simulink model "SVPWM_Combined"  (R2018b)
settings: Solver=FixedStepAuto  StartTime=0.0  StopTime=2000e-3  FixedStep=5e-7  RelTol=1e-3
libraries: powerlib x30, powerlib_meascontrol x5
settings Model: Creator=seogan  LastModifiedBy=Lenovo

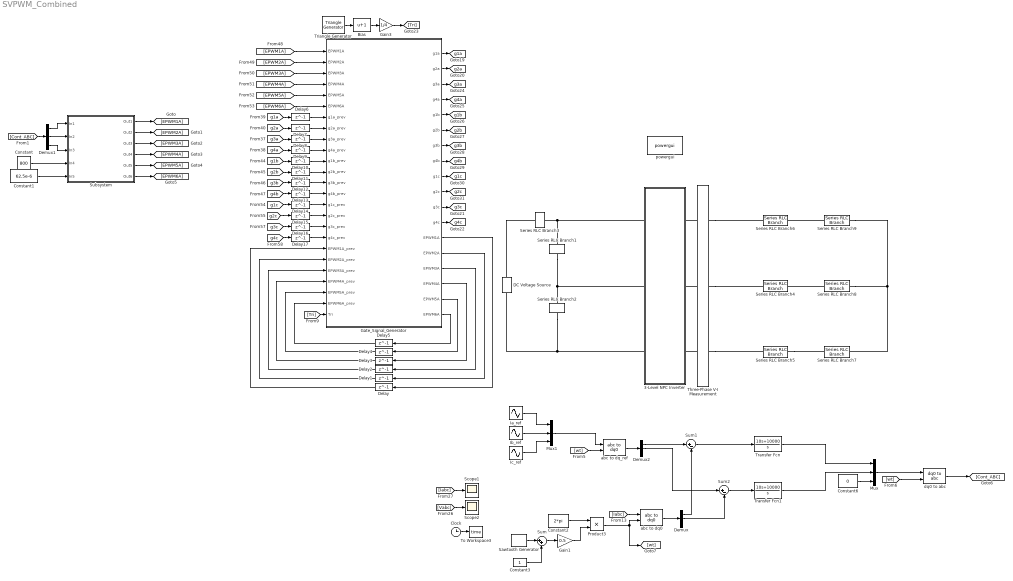
== system SVPWM_Combined ==
  3-Level NPC Inverter : Subsystem
  Bias : Bias  Bias=1
  Clock : Clock
  Constant : Constant  Value=800
  Constant1 : Constant  Value=62.5e-6
  Constant2 : Constant  Value=2*pi
  Constant3 : Constant
  Constant6 : Constant  Value=0
  DC Voltage Source : powerlib/Electrical Sources/DC Voltage Source  Amplitude=800  Measurements=None
  Delay{,1..17} (18 alike) : Delay  DelayLength=1
  Demux : Demux  Outputs=3
  Demux1 : Demux  Outputs=3
  Demux2 : Demux  Outputs=3
  Gain1 : Gain  Gain=0.5
  Gain3 : Gain  Gain=1/4
  Gate_Signal_Generator : MATLAB Function  TreatAsAtomicUnit=on
  Ia_ref : Sin  Amplitude=87.4  Frequency=50*2*pi  Phase=-62*pi/180  SampleTime=0
  Ib_ref : Sin  Amplitude=87.4  Frequency=50*2*pi  Phase=-62*pi/180-2*pi/3  SampleTime=0
  Ic_ref : Sin  Amplitude=87.4  Frequency=50*2*pi  Phase=-62*pi/180-4*pi/3  SampleTime=0
  Mux : Mux  Inputs=3
  Mux1 : Mux  Inputs=3
  Product3 : Product
  Sawtooth Generator : powerlib_meascontrol/Pulse & Signal Generators/Sawtooth Generator  Freq=50  Phase=0  Ts=5e-7
      settings: SourceProductName=Simscape Power Systems
  Scope1 : Scope
  Scope2 : Scope
  Series RLC Branch1 : powerlib/Elements/Series RLC Branch  LConnTagsString=__new0  RConnTagsString=__new0  BranchType=C  Resistance=1e-3  Inductance=1e-3  SetiL0=off  InitialCurrent=0  Capacitance=500e-6  Setx0=on  InitialVoltage=800/2  Measurements=Branch voltage
  Series RLC Branch2 : powerlib/Elements/Series RLC Branch  LConnTagsString=__new0  RConnTagsString=__new0  BranchType=C  Resistance=1e-3  Inductance=1e-3  SetiL0=off  InitialCurrent=0  Capacitance=500e-6  Setx0=on  InitialVoltage=800/2  Measurements=None
  Series RLC Branch3 : powerlib/Elements/Series RLC Branch  LConnTagsString=__new0  RConnTagsString=__new0  BranchType=R  Resistance=1e-3  Inductance=10e-3  SetiL0=on  InitialCurrent=88  Capacitance=1e-6  Setx0=off  InitialVoltage=0  Measurements=None
  Series RLC Branch4 : powerlib/Elements/Series RLC Branch  LConnTagsString=__new0  RConnTagsString=__new0  BranchType=R  Resistance=0.1  Inductance=0.6e-3  SetiL0=off  InitialCurrent=0  Capacitance=1e-6  Setx0=off  InitialVoltage=0  Measurements=None
  Series RLC Branch5 : powerlib/Elements/Series RLC Branch  LConnTagsString=__new0  RConnTagsString=__new0  BranchType=R  Resistance=0.1  Inductance=0.6e-3  SetiL0=off  InitialCurrent=0  Capacitance=1e-6  Setx0=off  InitialVoltage=0  Measurements=None
  Series RLC Branch6 : powerlib/Elements/Series RLC Branch  LConnTagsString=__new0  RConnTagsString=__new0  BranchType=R  Resistance=0.1  Inductance=0.6e-3  SetiL0=off  InitialCurrent=0  Capacitance=1e-6  Setx0=off  InitialVoltage=0  Measurements=None
  Series RLC Branch7 : powerlib/Elements/Series RLC Branch  LConnTagsString=__new0  RConnTagsString=__new0  BranchType=L  Resistance=0.1  Inductance=0.6e-3  SetiL0=off  InitialCurrent=0  Capacitance=1e-6  Setx0=off  InitialVoltage=0  Measurements=None
  Series RLC Branch8 : powerlib/Elements/Series RLC Branch  LConnTagsString=__new0  RConnTagsString=__new0  BranchType=L  Resistance=0.1  Inductance=0.6e-3  SetiL0=off  InitialCurrent=0  Capacitance=1e-6  Setx0=off  InitialVoltage=0  Measurements=None
  Series RLC Branch9 : powerlib/Elements/Series RLC Branch  LConnTagsString=__new0  RConnTagsString=__new0  BranchType=L  Resistance=0.1  Inductance=0.6e-3  SetiL0=off  InitialCurrent=0  Capacitance=1e-6  Setx0=off  InitialVoltage=0  Measurements=None
  Subsystem : Subsystem
  Sum : Sum  Inputs=|++
  Sum1 : Sum  Inputs=|+-
  Sum2 : Sum  Inputs=|+-
  Three-Phase V-I Measurement : powerlib/Measurements/Three-Phase V-I Measurement  VoltageMeasurement=phase-to-phase  SetLabelV=on  LabelV=Vabc  Vpu=off  VpuLL=off  CurrentMeasurement=yes  SetLabelI=on  LabelI=Iabc  Ipu=off  Pbase=100e6  Vbase=500e3  OutputType=Complex  PhasorSimulation=off  PSBequivalent=0
  To Workspace3 : ToWorkspace  VariableName=time  SampleTime=-1
  Transfer Fcn : TransferFcn  Numerator=[10 10000]  Denominator=[1 0]
  Transfer Fcn1 : TransferFcn  Numerator=[10 10000]  Denominator=[1 0]
  Triangle Generator : powerlib_meascontrol/Pulse & Signal Generators/Triangle Generator  Freq=16e3  Phase=0  Ts=5e-7
  abc to dq0 : powerlib_meascontrol/Transformations/abc to dq0  Alignment=90 degrees behind phase A axis
  abc to dq_ref : powerlib_meascontrol/Transformations/abc to dq0  Alignment=90 degrees behind phase A axis
  dq0 to abc : powerlib_meascontrol/Transformations/dq0 to abc  Alignment=90 degrees behind phase A axis
  powergui : powerlib/powergui  Priority=1  SimulationMode=Discrete  SampleTime=500e-9  frequency=60  Iterations=50  frequencyindice=0  Pbase=100e6  ErrMax=1e-4  UnitsV=kV  UnitsW=MW  buscounter=0  FunctionMessages=off  echomessages=off  EnableUseOfTLC=off  CurrentSourceSwitches=off  DisableSnubberDevices=off  DisableRonSwitches=off  DisableVfSwitches=off  DisplayEquations=off  SolverType=Tustin/Backward Euler (TBE)  Interpol=off  ExternalGateDelay=off  methode=off  Ts=100  x0status=blocks  SPID=off  SwTol=0  HookPort=off  RestoreLinks=warning  ResistiveCurrentMeasurement=off  Frange=[0:2:500]  Ylog=off  Xlog=on  ShowGrid=off  save=off  variable=ZData  structure=0  ZoomFFT=off  StartTime=0.0  cycles=1  DisplayStyle=1  fundamental=60  FreqAxis=off  MaxFrequency=1000  frequencyindicesteady=1  RmsSteady=1  display=off
  tag scope: g1a=global, g1b=global, g1c=global, g2a=global, g2b=global, g2c=global, g3a=global, g3b=global, g3c=global, g4a=global, g4b=global, g4c=global
  wires:
  Clock/1 -> To Workspace3/1
  Gate_Signal_Generator/8(g4b) -> [g4b]
  [EPWM3A] -> Gate_Signal_Generator/3("EPWM3A ")
  Delay2/1 -> Gate_Signal_Generator/21(EPWM3A_prev)
  Gate_Signal_Generator/5(g1b) -> [g1b]
  Gate_Signal_Generator/18(EPWM6A) -> Delay5/1
  Gain3/1 -> [Tri]
  Gate_Signal_Generator/7(g3b) -> [g3b]
  Gate_Signal_Generator/16(EPWM4A) -> Delay3/1
  Gate_Signal_Generator/15(EPWM3A) -> Delay2/1
  Gate_Signal_Generator/4(g4a) -> [g4a]
  Gate_Signal_Generator/3(g3a) -> [g3a]
  Gate_Signal_Generator/14(EPWM2A) -> Delay1/1
  [EPWM5A] -> Gate_Signal_Generator/5("EPWM5A ")
  [EPWM2A] -> Gate_Signal_Generator/2("EPWM2A ")
  [EPWM6A] -> Gate_Signal_Generator/6("EPWM6A ")
  Gate_Signal_Generator/13(EPWM1A) -> Delay/1
  [EPWM4A] -> Gate_Signal_Generator/4("EPWM4A ")
  Delay3/1 -> Gate_Signal_Generator/22(EPWM4A_prev)
  Gate_Signal_Generator/6(g2b) -> [g2b]
  [EPWM1A] -> Gate_Signal_Generator/1("EPWM1A ")
  Bias/1 -> Gain3/1
  Gate_Signal_Generator/9(g1c) -> [g1c]
  Gate_Signal_Generator/2(g2a) -> [g2a]
  Gate_Signal_Generator/11(g3c) -> [g3c]
  Delay5/1 -> Gate_Signal_Generator/24(EPWM6A_prev)
  Gate_Signal_Generator/10(g2c) -> [g2c]
  Delay4/1 -> Gate_Signal_Generator/23(EPWM5A_prev)
  Delay1/1 -> Gate_Signal_Generator/20(EPWM2A_prev)
  Gate_Signal_Generator/1(g1a) -> [g1a]
  Gate_Signal_Generator/12(g4c) -> [g4c]
  Gate_Signal_Generator/17(EPWM5A) -> Delay4/1
  Delay/1 -> Gate_Signal_Generator/19(EPWM1A_prev)
  [Tri] -> Gate_Signal_Generator/25(Tri)
  Triangle Generator/1 -> Bias/1
  Delay6/1 -> Gate_Signal_Generator/7(g1a_prev)
  [g1a] -> Delay6/1
  Delay7/1 -> Gate_Signal_Generator/8(g2a_prev)
  Delay8/1 -> Gate_Signal_Generator/9(g3a_prev)
  Delay9/1 -> Gate_Signal_Generator/10(g4a_prev)
  [g2a] -> Delay7/1
  [g3a] -> Delay8/1
  [g4a] -> Delay9/1
  Delay10/1 -> Gate_Signal_Generator/11(g1b_prev)
  Delay11/1 -> Gate_Signal_Generator/12(g2b_prev)
  Delay12/1 -> Gate_Signal_Generator/13(g3b_prev)
  Delay13/1 -> Gate_Signal_Generator/14(g4b_prev)
  [g1b] -> Delay10/1
  [g2b] -> Delay11/1
  [g3b] -> Delay12/1
  [g4b] -> Delay13/1
  Delay14/1 -> Gate_Signal_Generator/15(g1c_prev)
  Delay15/1 -> Gate_Signal_Generator/16(g2c_prev)
  Delay16/1 -> Gate_Signal_Generator/17(g3c_prev)
  Delay17/1 -> Gate_Signal_Generator/18(g4c_prev)
  [g1c] -> Delay14/1
  [g2c] -> Delay15/1
  [g3c] -> Delay16/1
  [g4c] -> Delay17/1
  [Vabc] -> Scope2/1
  [Iabc] -> Scope1/1
  Sawtooth Generator/1 -> Sum/1
  Constant3/1 -> Sum/2
  Sum/1 -> Gain1/1
  Gain1/1 -> Product3/2
  Constant2/1 -> Product3/1
  Product3/1 -> abc to dq0/2, [wt]
  Demux/1 -> Sum1/2
  Demux/2 -> Sum2/2
  Mux/1 -> dq0 to abc/1
  Constant6/1 -> Mux/3
  dq0 to abc/1 -> [Cont_ABC]
  [wt] -> abc to dq_ref/2
  Mux1/1 -> abc to dq_ref/1
  Ib_ref/1 -> Mux1/2
  Ia_ref/1 -> Mux1/1
  Ic_ref/1 -> Mux1/3
  abc to dq_ref/1 -> Demux2/1
  [wt] -> dq0 to abc/2
  abc to dq0/1 -> Demux/1
  Demux2/1 -> Sum1/1
  Demux2/2 -> Sum2/1
  [Iabc] -> abc to dq0/1
  Transfer Fcn/1 -> Mux/1
  Transfer Fcn1/1 -> Mux/2
  Sum1/1 -> Transfer Fcn/1
  Sum2/1 -> Transfer Fcn1/1
  Subsystem/6(Out6) -> [EPWM6A]
  Subsystem/1(Out1) -> [EPWM1A]
  Constant/1 -> Subsystem/4(In4)
  Subsystem/4(Out4) -> [EPWM4A]
  Subsystem/2(Out2) -> [EPWM2A]
  Subsystem/5(Out5) -> [EPWM5A]
  Constant1/1 -> Subsystem/5(In5)
  Subsystem/3(Out3) -> [EPWM3A]
  [Cont_ABC] -> Demux1/1
  Demux1/1 -> Subsystem/1(In1)
  Demux1/2 -> Subsystem/2(In2)
  Demux1/3 -> Subsystem/3(In3)
  connections:
  DC Voltage Source/LConn1 -- Series RLC Branch2/RConn1 -- 3-Level NPC Inverter/LConn3
  Three-Phase V-I Measurement/LConn3 -- 3-Level NPC Inverter/RConn3
  Three-Phase V-I Measurement/LConn2 -- 3-Level NPC Inverter/RConn2
  Three-Phase V-I Measurement/LConn1 -- 3-Level NPC Inverter/RConn1
  3-Level NPC Inverter/LConn2 -- Series RLC Branch1/RConn1 -- Series RLC Branch2/LConn1
  Series RLC Branch1/LConn1 -- 3-Level NPC Inverter/LConn1 -- Series RLC Branch3/RConn1
  DC Voltage Source/RConn1 -- Series RLC Branch3/LConn1
  Series RLC Branch8/LConn1 -- Series RLC Branch4/RConn1
  Series RLC Branch9/LConn1 -- Series RLC Branch6/RConn1
  Series RLC Branch5/RConn1 -- Series RLC Branch7/LConn1
  Series RLC Branch9/RConn1 -- Series RLC Branch7/RConn1 -- Series RLC Branch8/RConn1
  Three-Phase V-I Measurement/RConn1 -- Series RLC Branch6/LConn1
  Three-Phase V-I Measurement/RConn2 -- Series RLC Branch4/LConn1
  Three-Phase V-I Measurement/RConn3 -- Series RLC Branch5/LConn1

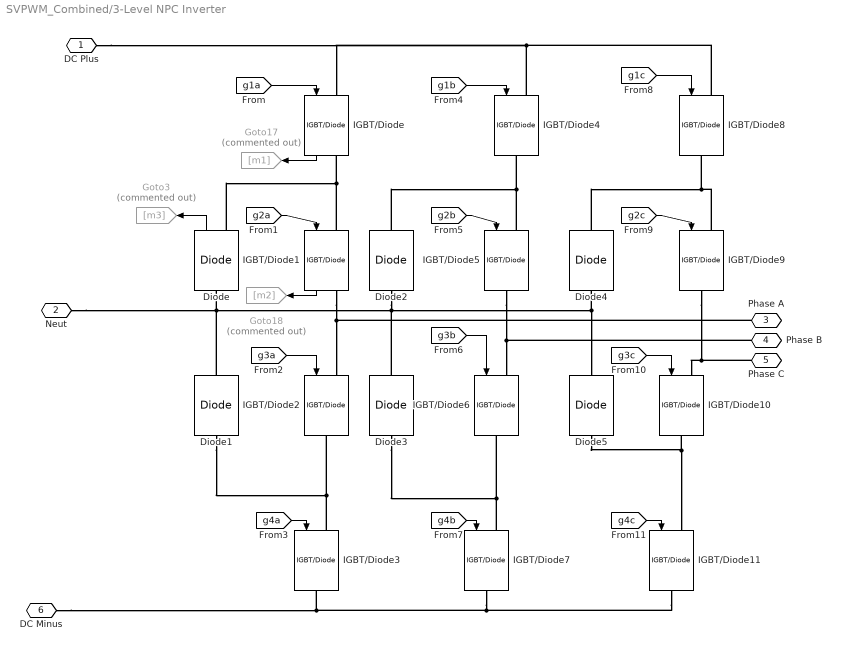
== system SVPWM_Combined/3-Level NPC Inverter ==
  Diode : powerlib/Power Electronics/Diode  Ron=1e-5  Lon=0  Vf=0.8  IC=0  UseSnubber=0  Rs=1e6  Cs=inf  Measurements=on
  Diode{1..5} (5 alike) : powerlib/Power Electronics/Diode  Ron=1e-5  Lon=0  Vf=0.8  IC=0  UseSnubber=0  Rs=1e6  Cs=inf  Measurements=off
  Goto17 : Goto  Commented=on  GotoTag=m1
  Goto18 : Goto  Commented=on  GotoTag=m2
  Goto3 : Goto  Commented=on  GotoTag=m3
  IGBT/Diode : powerlib/Power Electronics/IGBT//Diode  Ron=1e-3  Rs=1e3  Cs=inf  Measurements=on
  IGBT/Diode1 : powerlib/Power Electronics/IGBT//Diode  Ron=1e-3  Rs=1e3  Cs=inf  Measurements=on
  IGBT/Diode{2..11} (10 alike) : powerlib/Power Electronics/IGBT//Diode  Ron=1e-3  Rs=1e3  Cs=inf  Measurements=off
  DC Plus : PMIOPort  Side=Left
  " Neut" : PMIOPort  Port=2  Side=Left
  Phase A : PMIOPort  Port=3  Side=Right
  Phase B : PMIOPort  Port=4  Side=Right
  Phase C : PMIOPort  Port=5  Side=Right
  DC Minus : PMIOPort  Port=6  Side=Left
  wires:
  [g1a] -> IGBT/Diode/1
  [g3a] -> IGBT/Diode2/1
  [g2b] -> IGBT/Diode5/1
  [g3b] -> IGBT/Diode6/1
  [g4b] -> IGBT/Diode7/1
  [g2c] -> IGBT/Diode9/1
  [g3c] -> IGBT/Diode10/1
  [g4c] -> IGBT/Diode11/1
  [g4a] -> IGBT/Diode3/1
  [g1b] -> IGBT/Diode4/1
  [g1c] -> IGBT/Diode8/1
  [g2a] -> IGBT/Diode1/1
  IGBT/Diode/1 -> Goto17/1
  IGBT/Diode1/1 -> Goto18/1
  Diode/1 -> Goto3/1
  connections:
  IGBT/Diode11/RConn1 -- IGBT/Diode7/RConn1 -- DC Minus/RConn1 -- IGBT/Diode3/RConn1
  IGBT/Diode1/LConn1 -- IGBT/Diode/RConn1 -- Diode/RConn1
  IGBT/Diode9/RConn1 -- Phase C/RConn1 -- IGBT/Diode10/LConn1
  IGBT/Diode5/RConn1 -- Phase B/RConn1 -- IGBT/Diode6/LConn1
  IGBT/Diode7/LConn1 -- Diode3/LConn1 -- IGBT/Diode6/RConn1
  IGBT/Diode1/RConn1 -- Phase A/RConn1 -- IGBT/Diode2/LConn1
  IGBT/Diode5/LConn1 -- Diode2/RConn1 -- IGBT/Diode4/RConn1
  IGBT/Diode3/LConn1 -- Diode1/LConn1 -- IGBT/Diode2/RConn1
  IGBT/Diode9/LConn1 -- Diode4/RConn1 -- IGBT/Diode8/RConn1
  Diode1/RConn1 -- Diode3/RConn1 -- Diode5/RConn1 -- Diode4/LConn1 -- Diode2/LConn1 -- " Neut"/RConn1 -- Diode/LConn1
  DC Plus/RConn1 -- IGBT/Diode/LConn1 -- IGBT/Diode8/LConn1 -- IGBT/Diode4/LConn1
  Diode5/LConn1 -- IGBT/Diode11/LConn1 -- IGBT/Diode10/RConn1

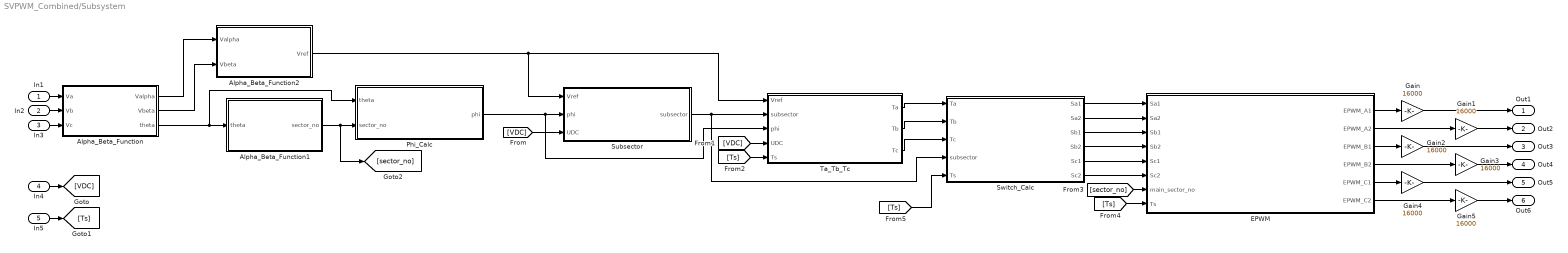
== system SVPWM_Combined/Subsystem ==
  In1 : Inport
  In2 : Inport  Port=2
  In3 : Inport  Port=3
  In4 : Inport  Port=4
  In5 : Inport  Port=5
  Alpha_Beta_Function : MATLAB Function  TreatAsAtomicUnit=on
  Alpha_Beta_Function1 : MATLAB Function  TreatAsAtomicUnit=on
  Alpha_Beta_Function2 : MATLAB Function  TreatAsAtomicUnit=on
  EPWM : MATLAB Function  TreatAsAtomicUnit=on
  Gain{,1..5} (6 alike) : Gain  Gain=16000
  Phi_Calc : MATLAB Function  TreatAsAtomicUnit=on
  Subsector : MATLAB Function  TreatAsAtomicUnit=on
  Switch_Calc : MATLAB Function  TreatAsAtomicUnit=on
  Ta_Tb_Tc : MATLAB Function  TreatAsAtomicUnit=on
  Out1 : Outport
  Out2 : Outport  Port=2
  Out3 : Outport  Port=3
  Out4 : Outport  Port=4
  Out5 : Outport  Port=5
  Out6 : Outport  Port=6
  wires:
  Ta_Tb_Tc/1(Ta) -> Switch_Calc/1(Ta)
  [Ts] -> Switch_Calc/5(Ts)
  Alpha_Beta_Function/3(theta) -> Phi_Calc/1(theta), Alpha_Beta_Function1/1(theta)
  Switch_Calc/1(Sa1) -> EPWM/1(Sa1)
  [Ts] -> EPWM/8(Ts)
  Subsector/1(subsector) -> Switch_Calc/4(subsector), Ta_Tb_Tc/2(subsector)
  Alpha_Beta_Function/1(Valpha) -> Alpha_Beta_Function2/1(Valpha)
  [VDC] -> Ta_Tb_Tc/4(UDC)
  EPWM/2(EPWM_A2) -> Gain1/1
  [VDC] -> Subsector/3(UDC)
  Phi_Calc/1(phi) -> Ta_Tb_Tc/3(phi), Subsector/2(phi)
  Ta_Tb_Tc/3(Tc) -> Switch_Calc/3(Tc)
  EPWM/5(EPWM_C1) -> Gain4/1
  [sector_no] -> EPWM/7(main_sector_no)
  [Ts] -> Ta_Tb_Tc/5(Ts)
  Ta_Tb_Tc/2(Tb) -> Switch_Calc/2(Tb)
  Switch_Calc/6(Sc2) -> EPWM/6(Sc2)
  Switch_Calc/5(Sc1) -> EPWM/5(Sc1)
  Alpha_Beta_Function1/1(sector_no) -> [sector_no], Phi_Calc/2(sector_no)
  Switch_Calc/3(Sb1) -> EPWM/3(Sb1)
  Switch_Calc/2(Sa2) -> EPWM/2(Sa2)
  Alpha_Beta_Function/2(Vbeta) -> Alpha_Beta_Function2/2(Vbeta)
  In5/1 -> [Ts]
  In2/1 -> Alpha_Beta_Function/2(Vb)
  EPWM/6(EPWM_C2) -> Gain5/1
  Alpha_Beta_Function2/1(Vref) -> Ta_Tb_Tc/1(Vref), Subsector/1(Vref)
  EPWM/3(EPWM_B1) -> Gain2/1
  Switch_Calc/4(Sb2) -> EPWM/4(Sb2)
  EPWM/4(EPWM_B2) -> Gain3/1
  EPWM/1(EPWM_A1) -> Gain/1
  In3/1 -> Alpha_Beta_Function/3(Vc)
  In1/1 -> Alpha_Beta_Function/1(Va)
  In4/1 -> [VDC]
  Gain/1 -> Out1/1
  Gain1/1 -> Out2/1
  Gain2/1 -> Out3/1
  Gain3/1 -> Out4/1
  Gain4/1 -> Out5/1
  Gain5/1 -> Out6/1

== matlab function SVPWM_Combined/Subsystem/Alpha_Beta_Function ==
  data: Va input; Valpha output; Vb input; Vc input; Vbeta output; theta output
function [Valpha, Vbeta, theta] = fcn(Va, Vb, Vc)
Valpha=2/3*Va-Vb/3-Vc/3;
Vbeta=Vb/sqrt(3)-Vc/sqrt(3);
theta=atan2(Vbeta,Valpha);
end

== matlab function SVPWM_Combined/Subsystem/Alpha_Beta_Function1 ==
  data: theta input; sector_no output
function sector_no = fcn(theta)
sector_no=0;
if (theta>=0) && (theta<pi/3)
    sector_no=1;
end
if (theta>=pi/3) && (theta<2*pi/3)
    sector_no=2;
end
if (theta>=2*pi/3) && (theta<pi)
    sector_no=3;
end
if (theta>=-pi/3) && (theta<0)
    sector_no=6;
end
if (theta>=-2*pi/3) && (theta<-pi/3)
    sector_no=5;
end
if (theta>=-pi) && (theta<-2*pi/3)
    sector_no=4;
end
end

== matlab function SVPWM_Combined/Subsystem/Phi_Calc ==
  data: theta input; phi output; sector_no input
function phi = fcn(theta, sector_no)
phi=0;
if (sector_no==1)
    phi=theta;
end

if (sector_no==2)
    phi=theta-pi/3;
end

if (sector_no==3)
    phi=theta-2*pi/3;
end

if (sector_no==6)
    phi=theta+pi/3;
end

if (sector_no==5)
    phi=theta+2*pi/3;
end

if (sector_no==4)
    phi=theta+pi;
end
end

== matlab function SVPWM_Combined/Subsystem/Alpha_Beta_Function2 ==
  data: Valpha input; Vref output; Vbeta input
function Vref = fcn(Valpha, Vbeta)
Vref=sqrt(Valpha^2+Vbeta^2);

== matlab function SVPWM_Combined/Subsystem/Subsector ==
  data: Vref input; subsector output; phi input; UDC input
function subsector = fcn(Vref, phi, UDC)
subsector=0;
n=Vref/(2/3*UDC);
m1=n*2/sqrt(3)*(sin(pi/3-phi));
m2=n*2/sqrt(3)*sin(phi);
if (m1<0.5) && (m2<0.5) && (m1+m2<0.5)
    subsector=1;
end
if (m1<0.5) && (m2<0.5) && (m1+m2>0.5)
    subsector=2;
end
if (m1>0.5)
    subsector=4;
end
if (m2>0.5)
    subsector=3;
end

end

== matlab function SVPWM_Combined/Subsystem/Ta_Tb_Tc ==
  data: Vref input; subsector input; Ta output; phi input; UDC input; Ts input; Tb output; Tc output
function [Ta, Tb, Tc] = fcn(Vref, subsector, phi, UDC, Ts)
Ta=0; 
Tb=0; 
Tc=0;

m=Vref/(2/3*UDC);
k=2/sqrt(3)*m*Ts;

if (subsector==1)
        Ta=2*k*sin(pi/3-phi);
        Tb=Ts-2*k*sin(pi/3+phi);
        Tc=2*k*sin(phi);
end
if (subsector==2)
        Ta=Ts-2*k*sin(phi);
        Tb=2*k*sin(pi/3+phi)-Ts;
        Tc=Ts-2*k*sin(pi/3-phi);
end
if (subsector==3)
        Ta=2*k*sin(phi)-Ts;
        Tb=2*k*sin(pi/3-phi);
        Tc=2*Ts-2*k*sin(pi/3+phi);
end
if (subsector==4)
        Ta=2*Ts-2*k*sin(pi/3+phi);
        Tb=2*k*sin(phi);
        Tc=2*k*sin(pi/3-phi)-Ts;
end

end

== matlab function SVPWM_Combined/Subsystem/Switch_Calc ==
  data: Ta input; Tb input; Sa1 output; Tc input; Sa2 output; Sb1 output; Sb2 output; Sc1 output; Sc2 output; subsector input; Ts input
function [Sa1, Sa2, Sb1, Sb2, Sc1, Sc2] = fcn(Ta, Tb, Tc, subsector, Ts)
Sa1=0; Sa2=0;
Sb1=0; Sb2=0;
Sc1=0; Sc2=0;

if (subsector==1)
       Sa1=(Tc+Ta)/4;
       Sa2=Ts/2;
       Sb1=Tc/4;
       Sb2=Ts/2-Ta/4;
       Sc1=0;
       Sc2=Ts/2-Ta/4-Tc/4;
end
if (subsector==2)
       Sa1=(Ta+Tc)/4+Tb/2;
       Sa2=Ts/2;
       Sb1=Tc/4;
       Sb2=Ts/2-Ta/4;
       Sc1=0;
       Sc2=(Ta+Tc)/4;
end
if (subsector==3)
       Sa1=Ts/2-Tc/4;
       Sa2=Ts/2;
       Sb1=Ta/2+Tc/4;
       Sb2=Ts/2;
       Sc1=0;
       Sc2=Tc/4;
end
if (subsector==4)
       Sa1=Ts/2-Ta/4;
       Sa2=Ts/2;
       Sb1=0;
       Sb2=Ta/4+Tb/2;
       Sc1=0;
       Sc2=Ta/4;
end
end

== matlab function SVPWM_Combined/Subsystem/EPWM ==
  data: Sa1 input; Sa2 input; EPWM_A1 output; Sb1 input; EPWM_A2 output; EPWM_B1 output; EPWM_B2 output; EPWM_C1 output; EPWM_C2 output; Sb2 input; Sc1 input; Sc2 input; main_sector_no input; Ts input
function [EPWM_A1, EPWM_A2, EPWM_B1, EPWM_B2, EPWM_C1, EPWM_C2] = fcn(Sa1, Sa2, Sb1, Sb2, Sc1, Sc2, main_sector_no, Ts)
EPWM_A1=0; EPWM_A2=0;
EPWM_B1=0; EPWM_B2=0;
EPWM_C1=0; EPWM_C2=0;


if (main_sector_no==1)
        EPWM_A1=Sa1; EPWM_A2=Sa2;
        EPWM_B1=Sb1; EPWM_B2=Sb2;
        EPWM_C1=Sc1; EPWM_C2=Sc2;
end
if (main_sector_no==2)
        EPWM_A1=Ts/2-Sb2; EPWM_A2=Ts/2-Sb1;
        EPWM_B1=Ts/2-Sc2; EPWM_B2=Ts/2-Sc1;
        EPWM_C1=Ts/2-Sa2; EPWM_C2=Ts/2-Sa1;
end
if (main_sector_no==3)
        EPWM_A1=Sc1; EPWM_A2=Sc2;
        EPWM_B1=Sa1; EPWM_B2=Sa2;
        EPWM_C1=Sb1; EPWM_C2=Sb2;
end
if (main_sector_no==4)
        EPWM_A1=Ts/2-Sa2; EPWM_A2=Ts/2-Sa1;
        EPWM_B1=Ts/2-Sb2; EPWM_B2=Ts/2-Sb1;
        EPWM_C1=Ts/2-Sc2; EPWM_C2=Ts/2-Sc1;    
end
if (main_sector_no==5)
        EPWM_A1=Sb1; EPWM_A2=Sb2;
        EPWM_B1=Sc1; EPWM_B2=Sc2;
        EPWM_C1=Sa1; EPWM_C2=Sa2;
end
if (main_sector_no==6)
        EPWM_A1=Ts/2-Sc2; EPWM_A2=Ts/2-Sc1;
        EPWM_B1=Ts/2-Sa2; EPWM_B2=Ts/2-Sa1;
        EPWM_C1=Ts/2-Sb2; EPWM_C2=Ts/2-Sb1;
end
end

== matlab function SVPWM_Combined/Gate_Signal_Generator ==
  data: EPWM1A input; EPWM2A input; EPWM3A input; EPWM4A input; EPWM5A input; EPWM6A input; g1a_prev input; g2a_prev input; g3a_prev input; g4a_prev input; g1b_prev input; g2b_prev input; g3b_prev input; g4b_prev input; g1c_prev input; g2c_prev input; g3c_prev input; g4c_prev input; EPWM1A_prev input; EPWM2A_prev input; EPWM3A_prev input; EPWM4A_prev input; EPWM5A_prev input; EPWM6A_prev input; g1a output; g2a output; g3a output; g4a output; g1b output; g2b output; g3b output; g4b output; g1c output; g2c output; g3c output; g4c output; Tri input; EPWM1A output; EPWM2A output; EPWM3A output; EPWM4A output; EPWM5A output; EPWM6A output
function [g1a,g2a,g3a,g4a,g1b,g2b,g3b,g4b,g1c,g2c,g3c,g4c,EPWM1A,EPWM2A,EPWM3A,EPWM4A,EPWM5A,EPWM6A] = fcn(EPWM1A,EPWM2A,EPWM3A,EPWM4A,EPWM5A,EPWM6A,g1a_prev,g2a_prev,g3a_prev,g4a_prev,g1b_prev,g2b_prev,g3b_prev,g4b_prev,g1c_prev,g2c_prev,g3c_prev,g4c_prev,EPWM1A_prev,EPWM2A_prev,EPWM3A_prev,EPWM4A_prev,EPWM5A_prev,EPWM6A_prev,Tri)
if(Tri>0.001)
    EPWM1A=EPWM1A_prev;
    EPWM2A=EPWM2A_prev;
    EPWM3A=EPWM3A_prev;
    EPWM4A=EPWM4A_prev;
    EPWM5A=EPWM5A_prev;
    EPWM6A=EPWM6A_prev;
end
    g1a=g1a_prev;
    g3a=g3a_prev;
    g2a=g2a_prev;
    g4a=g4a_prev;
    g1b=g1b_prev;
    g3b=g3b_prev;
    g2b=g2b_prev;
    g4b=g4b_prev;
    g1c=g1c_prev;
    g3c=g3c_prev;
    g2c=g2c_prev;
    g4c=g4c_prev;

if(Tri<EPWM1A)
    g1a=1;
    g3a=0;
end
if(Tri>=EPWM1A)
    g1a=0;
    g3a=1;
end

if(Tri<EPWM2A)
    g2a=1;
    g4a=0;
end
if(Tri>=EPWM2A)
    g2a=0;
    g4a=1;
end
if(Tri<EPWM3A)
    g1b=1;
    g3b=0;
end
if(Tri>=EPWM3A)
    g1b=0;
    g3b=1;
end

if(Tri<EPWM4A)
    g2b=1;
    g4b=0;
end
if(Tri>=EPWM4A)
    g2b=0;
    g4b=1;
end

if(Tri<EPWM5A)
    g1c=1;
    g3c=0;
end
if(Tri>=EPWM5A)
    g1c=0;
    g3c=1;
end

if(Tri<EPWM6A)
    g2c=1;
    g4c=0;
end
if(Tri>=EPWM6A)
    g2c=0;
    g4c=1;
end

% if(Tri>EPWM1A)
%     g1a=1;
%     g3a=0;
% elseif(Tri<EPWM1A)
%     g1a=0;
%     g3a=1;
% else
%     g1a=g1a_prev;
%     g3a=g3a_prev;
% end
% 
% if(Tri>EPWM2A)
%     g2a=1;
%     g4a=0;
% elseif(Tri<EPWM2A)
%     g2a=0;
%     g4a=1;
% else
%     g2a=g2a_prev;
%     g4a=g4a_prev;
% end
% 
% if(Tri>EPWM3A)
%     g1b=1;
%     g3b=0;
% elseif(Tri<EPWM3A)
%     g1b=0;
%     g3b=1;
% else
%     g1b=g1b_prev;
%     g3b=g3b_prev;
% end
% 
% if(Tri>EPWM4A)
%     g2b=1;
%     g4b=0;
% elseif(Tri<EPWM4A)
%     g2b=0;
%     g4b=1;
% else
%     g2b=g2b_prev;
%     g4b=g4b_prev;
% end
% 
% if(Tri>EPWM5A)
%     g1c=1;
%     g3c=0;
% elseif(Tri<EPWM5A)
%     g1c=0;
%     g3c=1;
% else
%     g1c=g1c_prev;
%     g3c=g3c_prev;
% end
% 
% if(Tri>EPWM6A)
%     g2c=1;
%     g4c=0;
% elseif(Tri<EPWM6A)
%     g2c=0;
%     g4c=1;
% else
%     g2c=g2c_prev;
%     g4c=g4c_prev;
% end
end
